simulink model "plant_1"  (R2017b)
settings: Solver=VariableStepAuto  StartTime=0.0  StopTime=10  FixedStep=10e-5
settings Model: Creator=Mehmet  LastModifiedBy=Mehmet

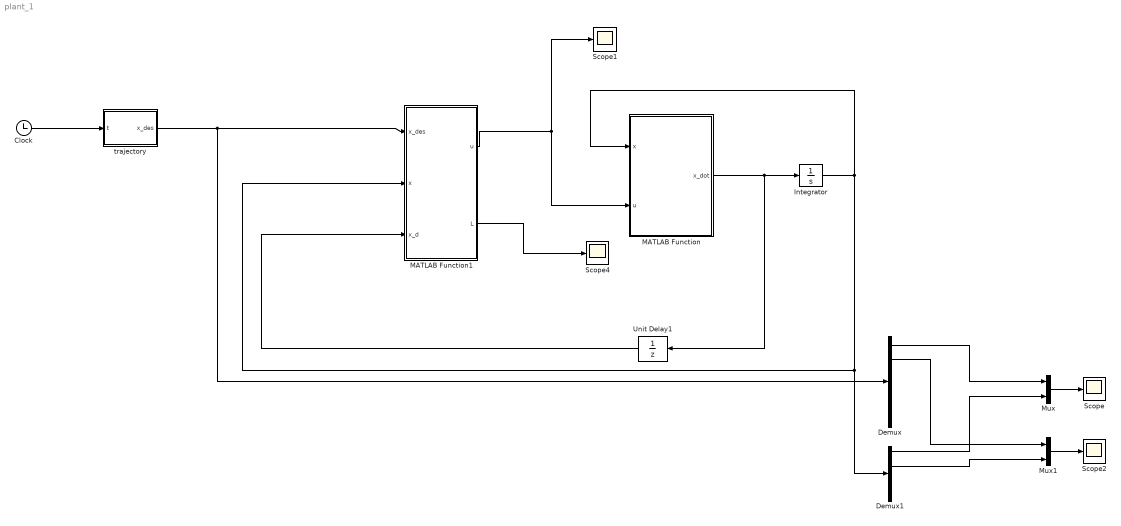
== system plant_1 ==
  Clock : Clock
  Demux : Demux  Outputs=6
  Demux1 : Demux
  Integrator : Integrator  InitialCondition=[0;0;0;0]
  MATLAB Function : MATLAB Function  TreatAsAtomicUnit=on
  MATLAB Function1 : MATLAB Function  TreatAsAtomicUnit=on
  Mux : Mux  Inputs=2
  Mux1 : Mux  Inputs=2
  Scope{,1..2,4} (4 alike) : Scope
  Unit Delay1 : UnitDelay  SampleTime=-1
  trajectory : MATLAB Function  TreatAsAtomicUnit=on
  wires:
  MATLAB Function1/1(u) -> MATLAB Function/2(u), Scope1/1
  Clock/1 -> trajectory/1(t)
  trajectory/1(x_des) -> MATLAB Function1/1(x_des), Demux/1
  Demux/1 -> Mux/1
  Demux1/1 -> Mux/2
  Mux/1 -> Scope/1
  MATLAB Function/1(x_dot) -> Unit Delay1/1, Integrator/1
  Integrator/1 -> MATLAB Function1/2(x), Demux1/1, MATLAB Function/1(x)
  Unit Delay1/1 -> MATLAB Function1/3(x_d)
  Mux1/1 -> Scope2/1
  Demux/2 -> Mux1/1
  Demux1/2 -> Mux1/2
  MATLAB Function1/2(L) -> Scope4/1

== matlab function plant_1/MATLAB Function1 ==
  data: x_des input; u output; L output; x input; x_d input
function [u,L]  = fcn(x_des,x,x_d)

% PD Computed-Torque control input
m1 = 0.8; 
m2 = 2.3; 
a1 = 1; 
a2 = 1; 
g= 9.81; % arm parameters
 
Kv = 20*eye(2); % controller parameters
lam = 5*eye(2);
gam = 1*eye(2);

% tracking errors
qd = x_des(1:2,1);
qdp = x_des(3:4,1);
qdpp = x_des(5:6,1);

e = qd - [x(1) x(2)]';
ep = qdp - [x(3) x(4)]';

r = ep + lam*e;

u = Kv*r;

L = 1/2*r'*r;


end

== matlab function plant_1/MATLAB Function ==
  data: x input; u input; x_dot output
function x_dot = fcn(x,u)

% arm parameters
m1 = 0.8; 
m2 = 2.3; 
a1 = 1; 
a2 = 1; 
g = 9.81;   

% inertia M(q) and nonlinear terms N(q,qdot)
M11= (m1 + m2)*a1^2 + m2*a2^2 + 2*m2*a1*a2*cos(x(2)) ;
M12= m2*a2^2 + m2*a1*a2*cos(x(2)) ;
M22= m2*a2^2 ;
N1= -m2*a1*a2*(2*x(3)*x(4) + x(4)^2)*sin(x(2)) ;
N1= N1 + (m1 + m2)*g*a1*cos(x(1)) + m2*g*a2*cos(x(1) + x(2));
N2= m2*a1*a2*x(3)^2*sin(x(2)) + m2*g*a2*cos(x(1) + x(2)) ;

% Inversion of M(q) (for large values of n, use least-squares)
det= M11*M22 - M12*M12 ;
MI11= M22/det ;
MI12= -M12/det ;
MI22= M11/det ;

tau = zeros(2,1);

tau = u;
%% control input
tau1 = tau(1,1);
tau2 = tau(2,1);

q = zeros(4,1);

q(1) = x(3);
q(2) = x(4);
q(3) = MI11*(-N1 + tau1) + MI12*(-N2 + tau2);
q(4) = MI12*(-N1 + tau1) + MI22*(-N2 + tau2);

x_dot = q;

end

== matlab function plant_1/trajectory ==
  data: t input; x_des output
function x_des = fcn(t)

% compute desired trajectory
period= 8 ; amp1= 1 ; amp2= 1 ;
fact= 2*pi/period;
sinf= sin(fact*t);
cosf= cos(fact*t);
qd= [amp1*sinf amp2*cosf];
qdp= fact*[amp1*cosf -amp2*sinf];
qdpp= -fact^2*qd;

x_des = [qd qdp qdpp]';

end
